simulink model "DAB_TPS"  (R2026a)
settings: Solver=VariableStepAuto  StopTime=1
libraries: ee_lib x20, nesl_utility x13, fl_lib x6
settings Model: Creator=EV5_1  LastModifiedBy=EV5_1

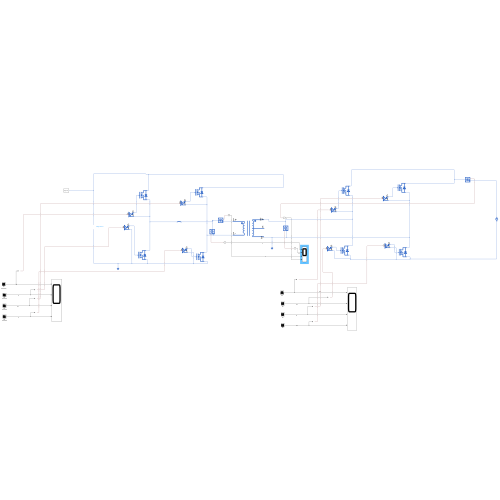
[thumbnail: Simulink's stored preview of the top-level diagram]
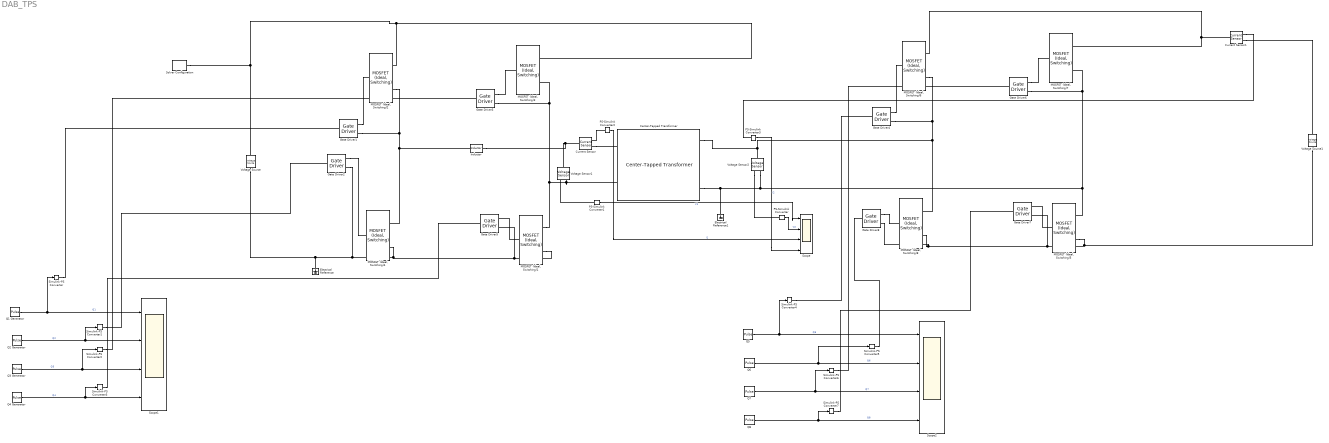
== system DAB_TPS ==
  Center-Tapped Transformer : ee_lib/Passive/Transformers/Center-Tapped Transformer  modeling_option=ee.enum.transformer_option.ideal  n=2  T=0.5  Rw1=0.01 Ohm  L1=0.0001 H  Rw2=0.01 Ohm  L2=0.0001 H  Rm=100 Ohm  Lm=0.04 H  i1_specify=off  i1_priority=None  i1=0 A  i1_nominal_specify=off  i1_nominal_value=1  i1_nominal_unit=A  i2p_specify=off  i2p_priority=None  i2p=0 A  i2p_nominal_specify=off  i2p_nominal_value=1  i2p_nominal_unit=A  i2n_specify=off  i2n_priority=None  i2n=0 A  i2n_nominal_specify=off  i2n_nominal_value=1  i2n_nominal_unit=A
  Current Sensor : fl_lib/Electrical/Electrical Sensors/Current Sensor
  Current Sensor1 : fl_lib/Electrical/Electrical Sensors/Current Sensor
  Electrical Reference : fl_lib/Electrical/Electrical Elements/Electrical Reference
  Electrical Reference1 : fl_lib/Electrical/Electrical Elements/Electrical Reference
  Gate Driver{1..8} (8 alike) : ee_lib/Semiconductors & Converters/Gate Driver  port_option=ee.enum.controlport.ps  uHigh=2.0 V  uLow=0.8 V  uHighValue=0.7  uLowValue=0.3  vHigh=15 V  vLow=0 V  tHigh=50 ns  tLow=50 ns  parameterization=ee.enum.semiconductors.gateDriverParam.outputImpedance  rHigh=2 Ohm  rLow=2 Ohm  tRise=20 ns  tFall=20 ns  cLoad=10 nF  ZonTime_specify=off  ZonTime_priority=None  ZonTime=0 s  ZoffTime_specify=off  ZoffTime_priority=None  ZoffTime=0 s
  Inductor : ee_lib/Passive/Inductor  l=3.88e-6 H  enable_L_tol=ee.enum.toleranceApplication.none  L_tol=20  tol_distribution=ee.enum.toleranceDistribution.uniform  nSigma=4  r=0 Ohm  g=1e-9 1/Ohm  enable_operating_limits=ee.enum.enable.no  operating_limit_action=ee.enum.passive.reportOpLim.warn  max_working_current=1 A  power_rating=1 W  i_L_specify=off  i_L_priority=High  i_L=0 A  i_L_nominal_specify=off  i_L_nominal_value=1  i_L_nominal_unit=A
  MOSFET (Ideal, Switching){1..8} (8 alike) : ee_lib/Semiconductors & Converters/MOSFET (Ideal, Switching)  port_option=ee.enum.controlport.elec  Rds=0.026 Ohm  Goff=1e-5 1/Ohm  Vth=3 V  diode_param=ee.enum.semiconductors.protectionDiode.chargedynamics  diode_Vf=1.3 V  diode_Ron=0.001 Ohm  diode_Goff=1e-5 1/Ohm  diode_C=1.36e-9 F  diode_iRM=-7.4 A  diode_iF=195 A  diode_idot=-100 A/us  diode_trr_param=ee.enum.converters.diodeReverseParam.trr_factor  diode_trr_factor=3  diode_trr=15 us  diode_Qrr=1500 s*uA  ids_specify=off  ids_priority=None  ids=0 A  ids_nominal_specify=off  ids_nominal_value=1  ids_nominal_unit=A  vds_specify=off  vds_priority=None  vds=0 V  vds_nominal_specify=off  vds_nominal_value=1  vds_nominal_unit=V  vgs_specify=off  vgs_priority=None  vgs=0 V  vgs_nominal_specify=off  vgs_nominal_value=1  vgs_nominal_unit=V  thermal_loss_option=ee.enum.converters.thermalLossOption.constantvalues  Von_data=[0, 1.8, 3.2, 6, 10, 16; 0, 2, 5.5, 9.5, 15, 25] V  Tj=[298.15, 448.15] K  Iout_data=[0, 20, 40, 60, 80, 100] A  tabulateWithVds=false  Eon_data=[0, 55.04, 124.57, 235.53, 362.12; 0, 71.25, 161.25, 304.88, 468.75] * 1e-6 J  Eoff_data=[0, 18, 30, 56.1, 76.5; 0, 22.5, 37.5, 70.13, 95.63] * 1e-6 J  Eon_data_3D=[zeros(2, 5, 3)] J  Eoff_data_3D=[zeros(2, 5, 3)] J  Tj_loss=[298.15, 448.15] K  Iout_data_loss=[0, 10, 20, 30, 40] A  Vds_loss=[0, 150, 300] V  Eon_scalar=22.86e-3 J  Eoff_scalar=17.14e-3 J  Voff=300 V  Iout_scalar=600 A  useCurrentFromPreviousCycle=false  useVoltageFromPreviousCycle=false  diodeModelType=ee.enum.converters.diodeModelType.pwl  diodeTableType=ee.enum.diode.tableType.IfMat  diode_ReverseIVType=ee.enum.diode.diodeReverseIV.constant  diode_IfMat=[.07, .12, .19, 1.75, 4.24, 7.32, 11.2; .16, .3, .72, 2.14, 4.02, 6.35, 9.12] A  diode_VfMat=[.9, 1.15, 1.25, 1.5, 1.75, 2.17, 2.6, 2.85; .58, .68, .75, 1.1, 1.38, 1.77, 2.27, 2.7] V  diode_TjVec=[25, 125] degC  diode_VfVec=[.5, .7, .9, 1.3, 1.7, 2.1, 2.5] V  diode_IfVec=[.1, .2, .5, 1, 2, 4, 7, 10] A  diode_IrMat=[1e-06, 2e-06, 5e-06, 1e-05, 2.5e-05, 5e-05, .0001; 2e-06, 5e-06, 1e-05, 4e-05, 8e-05, .0002, .0005] A  diode_VrMat=[10, 100, 200, 250, 300, 325, 350; 10, 70, 160, 220, 270, 300, 320] V  diode_VrVec=[10, 20, 40, 50, 70, 80, 100] V  diode_IrVec=[1e-06, 2e-06, 5e-06, 1e-05, 2e-05, 5e-05, .0001] A  diode_Vr=-600 V  diode_Ls=150 nH  diode_Erec=0.03 J  diode_rec_loss_model=ee.enum.diode.reverseRecoveryModelTabulateUpTo3D.fixed  diode_ErecVal=0 J  diode_scaleWithIandV=true  diode_ErecMat=zeros(2, 3) J  diodeErecMat3D=zeros(2, 3, 2) J  diode_TjrecVec=[298.15, 398.15] K  diode_IfrecVec=[.1, 1, 10] A  diodeVrecVec=[0, 100] V  diode_IrecVal=10 A  diode_VrecVal=10 V  diode_tFilter=1 / 1000 / 100 s  separateThermalPortForDiode=false  thermal_network_parameterization=ee.enum.thermalNetworkTopology.external  Rth=[.03, .2] K/W  Rth_Cauer=[.03, .1, .2] K/W  Rth_Foster=[.08, .14, .22, .16] K/W  thermal_mass_parameterization=ee.enum.thermalNetwork.timeconstant  thermal_mass=[3, 25] J/K  thermal_mass_Cauer=[3, 10, 25] J/K  thermal_mass_Foster=[.001, .005, .05, .5] J/K  thermal_time_constant=[.1, 5] s  thermal_time_constant_Cauer=[.1, 1, 5] s  thermal_time_constant_Foster=[7e-05, .0007, .01, .08] s  thermal_mass_initial_temperatures=[25, 25] degC  thermal_mass_initial_temperatures_Cauer=[25, 25, 25] degC  junction_thermal_mass=0.1 J/K  Tvec_initial_Foster=[25, 25, 25, 25] degC  RthDiode=[.03, .2] K/W  RthCauerDiode=[.03, .1, .2] K/W  RthFosterDiode=[.03, .2] K/W  thermalMassDiode=[3, 25] J/K  thermalMassCauerDiode=[3, 10, 25] J/K  thermalMassFosterDiode=[33, 50] J/K  thermalTauDiode=[.1, 5] s  thermalTauCauerDiode=[.1, 1, 5] s  thermalTauFosterDiode=[1, 10] s  thermalMassInitTempDiode=[25, 25] degC  thermalMassInitTempCauerDiode=[25, 25, 25] degC  junctionthermalMassDiode=0.1 J/K  TVecInitialFosterDiode=[25, 25, 25, 25] degC  no_thermal_network=ee.enum.enable.no  mosfet_junction_temperature_specify=off  mosfet_junction_temperature_priority=None  mosfet_junction_temperature=25 degC  mosfet_junction_temperature_nominal_specify=off  mosfet_junction_temperature_nominal_value=1  mosfet_junction_temperature_nominal_unit=degC  diode_junction_temperature_specify=off  diode_junction_temperature_priority=None  diode_junction_temperature=25 degC  diode_junction_temperature_nominal_specify=off  diode_junction_temperature_nominal_value=1  diode_junction_temperature_nominal_unit=degC  Qj_specify=off  Qj_priority=None  Qj=0 W  Qj_nominal_specify=off  Qj_nominal_value=1  Qj_nominal_unit=W  accumulatedSwitchingLosses_specify=off  accumulatedSwitchingLosses_priority=None  accumulatedSwitchingLosses=0 J
  PS-Simulink Converter{,1..3} (4 alike) : nesl_utility/PS-Simulink Converter  PhysicalDomain=network_engine_domain  SubClassName=ps_output  LeftPortType=input  RightPortType=output  PseudoPeriodic=off  Frequencies=[]  VectorFormat=inherit  Unit=inherit  AffineConversion=off
  Q1 Generator : DiscretePulseGenerator  PulseType=Time based  Amplitude=10  Period=1e-5  PulseWidth=45  PhaseDelay=1.25e-6
  Q2 Generator : DiscretePulseGenerator  PulseType=Time based  Amplitude=10  Period=1e-5  PulseWidth=50  PhaseDelay=6.25e-6
  Q3 Generator : DiscretePulseGenerator  PulseType=Time based  Amplitude=10  Period=1e-5  PulseWidth=45  PhaseDelay=3.75e-6
  Q4 Generator : DiscretePulseGenerator  PulseType=Time based  Amplitude=10  Period=1e-5  PulseWidth=45  PhaseDelay=8.75e-6
  Q5 : DiscretePulseGenerator  PulseType=Time based  Amplitude=10  Period=1e-5  PulseWidth=45  PhaseDelay=2.25e-6
  Q6 : DiscretePulseGenerator  PulseType=Time based  Amplitude=10  Period=1e-5  PulseWidth=45  PhaseDelay=7.25e-6
  Q7 : DiscretePulseGenerator  PulseType=Time based  Amplitude=10  Period=1e-5  PulseWidth=45  PhaseDelay=4.75e-6
  Q8 : DiscretePulseGenerator  PulseType=Time based  Amplitude=10  Period=1e-5  PulseWidth=50  PhaseDelay=9.75e-6
  Scope : Scope  NumInputPorts=4
      settings: ActiveDisplayYMinimum=-186.96880895174402  ActiveDisplayYMaximum=186.84605380979852
  Scope1 : Scope  NumInputPorts=4
      settings: ActiveDisplayYMinimum=-1.2499999999999998  ActiveDisplayYMaximum=11.25
  Scope2 : Scope  NumInputPorts=4
      settings: ActiveDisplayYMinimum=-1.2499999999999998  ActiveDisplayYMaximum=11.25  DataLoggingVariableName=ScopeData2
  Simulink-PS Converter{,1..7} (8 alike) : nesl_utility/Simulink-PS Converter  PhysicalDomain=network_engine_domain  SubClassName=ps_input  LeftPortType=input  RightPortType=output  PseudoPeriodic=off  Frequencies=[]  NoiseDistribution=none  NoiseParameters=[]  Unit=1  AffineConversion=off  FilteringAndDerivatives=provide  SimscapeFilterOrder=1  InputFilterTimeConstant=0.001  UdotUserProvided=0
  Solver Configuration : nesl_utility/Solver Configuration  PhysicalDomain=network_engine_domain  SubClassName=solver  LeftPortType=input  RightPortType=generic  Tones=[]  Harmonics=[]  SimulateNoise=off  Profile=off  UseLocalSampling=off  EnableSwitchedLinearOptims=on  FrequencyDomain=off  UseCCode=off  RelTol=0.001  AbsTol=0.001  MinStep=1e-09  ToWorkspace=off  RevertToSquareIcSolve=off  NumHomotopyIterations=100  PhasorMode=off  PhasorModeNumHarmonics=1  ConsistencySolver=NEWTON_XTOL_AFTER_FTOL  CanonicalOrdering=CANONICAL  OptimizeIntermediates=OPTIMIZED  IndexReductionMethod=DerivativeReplacement  DoDC=off  ResidualTolerance=1e-09  ConsistencyTolSource=GLOBAL  ConsistencyAbsTol=0.001  ConsistencyRelTol=0.001  ConsistencyTolFactor=0.001  UseLocalSolver=off  LocalSolverChoice=NE_BACKWARD_EULER_ADVANCER  ResolveIndetEquations=on  FunctionEvalNumThread=1  LocalSolverSampleTime=0.001  DoFixedCost=off  MaxNonlinIter=3  MaxModeIter=2  ComputeImpulses=off  ImpulseIterations=2  LinearAlgebra=auto  LinearAlgebraNumThread=0  EquationFormulation=NE_TIME_EF  DelaysMemoryBudget=1024  AutomaticFiltering=on  FilteringTimeConstant=0.001  PartitionStorageMethod=AS_NEEDED  PartitionMemoryBudget=1024  PartitionMethod=ROBUST  MultibodyUseLocalSolver=off  MultibodyLocalSolverChoice=ODE1  MultibodyLocalSolverSampleTime=0.001
  Voltage Sensor1 : fl_lib/Electrical/Electrical Sensors/Voltage Sensor
  Voltage Sensor2 : fl_lib/Electrical/Electrical Sensors/Voltage Sensor
  Voltage Source : ee_lib/Sources/Voltage Source  dc_voltage=36 V  ac_voltage=0 V  ac_shift=0 rad  ac_frequency=60 Hz  noise_mode=ee.enum.sources.noise.Disabled  PSD=0 V^2/Hz  sample_time=1e-3 s  repeatability=ee.enum.sources.repeatability.NotRepeatable  user_seed=0  auto_seed=3933054132  i_specify=off  i_priority=None  i=0 A  i_nominal_specify=off  i_nominal_value=1  i_nominal_unit=A  v_specify=off  v_priority=None  v=0 V  v_nominal_specify=off  v_nominal_value=1  v_nominal_unit=V
  Voltage Source1 : ee_lib/Sources/Voltage Source  dc_voltage=72 V  ac_voltage=0 V  ac_shift=0 rad  ac_frequency=60 Hz  noise_mode=ee.enum.sources.noise.Disabled  PSD=0 V^2/Hz  sample_time=1e-3 s  repeatability=ee.enum.sources.repeatability.NotRepeatable  user_seed=0  auto_seed=3402504572  i_specify=off  i_priority=None  i=0 A  i_nominal_specify=off  i_nominal_value=1  i_nominal_unit=A  v_specify=off  v_priority=None  v=0 V  v_nominal_specify=off  v_nominal_value=1  v_nominal_unit=V
  wires:
  Q1 Generator/1 -> Scope1/1, Simulink-PS Converter/1  "Q1"
  Q2 Generator/1 -> Simulink-PS Converter1/1, Scope1/2  "Q2"
  Q3 Generator/1 -> Simulink-PS Converter2/1, Scope1/3  "Q3"
  Q4 Generator/1 -> Simulink-PS Converter3/1, Scope1/4  "Q4"
  Q8/1 -> Simulink-PS Converter7/1, Scope2/4  "Q8"
  Q7/1 -> Simulink-PS Converter6/1, Scope2/3  "Q7"
  Q6/1 -> Simulink-PS Converter5/1, Scope2/2  "Q6"
  Q5/1 -> Scope2/1, Simulink-PS Converter4/1  "Q5"
  PS-Simulink Converter1/1 -> Scope/1  "V1"
  PS-Simulink Converter/1 -> Scope/2  "V2"
  PS-Simulink Converter2/1 -> Scope/3  "I1"
  PS-Simulink Converter3/1 -> Scope/4  "I2"
  connections:
  Gate Driver3/RConn2 -- "MOSFET (Ideal, Switching)3"/RConn2 -- Center-Tapped Transformer/LConn2 -- Voltage Sensor1/RConn2 -- "MOSFET (Ideal, Switching)1"/RConn1
  "MOSFET (Ideal, Switching)1"/RConn2 -- Electrical Reference/LConn1 -- Voltage Source/RConn1 -- Gate Driver2/RConn2 -- "MOSFET (Ideal, Switching)4"/RConn2 -- Gate Driver5/RConn2
  Gate Driver3/RConn1 -- "MOSFET (Ideal, Switching)3"/LConn1
  "MOSFET (Ideal, Switching)1"/LConn1 -- Gate Driver5/RConn1
  "MOSFET (Ideal, Switching)2"/RConn2 -- Gate Driver1/RConn2 -- "MOSFET (Ideal, Switching)4"/RConn1 -- Inductor/LConn1
  "MOSFET (Ideal, Switching)2"/RConn1 -- Solver Configuration/RConn1 -- Voltage Source/LConn1 -- "MOSFET (Ideal, Switching)3"/RConn1
  Gate Driver1/RConn1 -- "MOSFET (Ideal, Switching)2"/LConn1
  Gate Driver2/RConn1 -- "MOSFET (Ideal, Switching)4"/LConn1
  Simulink-PS Converter/RConn1 -- Gate Driver1/LConn1
  Simulink-PS Converter1/RConn1 -- Gate Driver2/LConn1
  Simulink-PS Converter2/RConn1 -- Gate Driver3/LConn1
  Simulink-PS Converter3/RConn1 -- Gate Driver5/LConn1
  PS-Simulink Converter1/LConn1 -- Voltage Sensor1/RConn1
  "MOSFET (Ideal, Switching)7"/RConn2 -- Gate Driver6/RConn2 -- Electrical Reference1/LConn1 -- Center-Tapped Transformer/RConn3 -- Voltage Sensor2/RConn2 -- "MOSFET (Ideal, Switching)5"/RConn1
  "MOSFET (Ideal, Switching)8"/RConn2 -- Gate Driver8/RConn2 -- Voltage Source1/RConn1 -- "MOSFET (Ideal, Switching)5"/RConn2 -- Gate Driver7/RConn2
  "MOSFET (Ideal, Switching)6"/RConn2 -- Gate Driver4/RConn2 -- Center-Tapped Transformer/RConn1 -- Voltage Sensor2/LConn1 -- "MOSFET (Ideal, Switching)8"/RConn1
  "MOSFET (Ideal, Switching)6"/RConn1 -- Current Sensor1/LConn1 -- "MOSFET (Ideal, Switching)7"/RConn1
  Gate Driver4/RConn1 -- "MOSFET (Ideal, Switching)6"/LConn1
  "MOSFET (Ideal, Switching)5"/LConn1 -- Gate Driver7/RConn1
  Gate Driver6/RConn1 -- "MOSFET (Ideal, Switching)7"/LConn1
  Simulink-PS Converter4/RConn1 -- Gate Driver4/LConn1
  Simulink-PS Converter5/RConn1 -- Gate Driver8/LConn1
  Gate Driver8/RConn1 -- "MOSFET (Ideal, Switching)8"/LConn1
  Simulink-PS Converter6/RConn1 -- Gate Driver6/LConn1
  Simulink-PS Converter7/RConn1 -- Gate Driver7/LConn1
  Voltage Sensor2/RConn1 -- PS-Simulink Converter/LConn1
  Current Sensor/RConn2 -- Center-Tapped Transformer/LConn1
  Current Sensor/RConn1 -- PS-Simulink Converter2/LConn1
  Current Sensor1/RConn1 -- PS-Simulink Converter3/LConn1
  Current Sensor/LConn1 -- Inductor/RConn1 -- Voltage Sensor1/LConn1
  Current Sensor1/RConn2 -- Voltage Source1/LConn1
